simulink model "mySimulationScheme"  (R2021a)
settings: Solver=VariableStepAuto  StartTime=0.0  StopTime=20  RelTol=1e-3
model workspace (MAT data in the model file):
  firstWarning = 1
  originalScenarioChecksum = 'C777D8D004E8227793BA6FB88E4AFE4A'
values from neighbouring files (symbols this model uses):
  A = [0 1 0;0 0 1;0 0 (-1/tau)]    [main.m]
  C = [0 1 0]    [main.m]
  h = 1    [main.m]
  lambda = 50    [main.m]
  Ts = 0.1    [main.m]
undefined symbols (not defined in the file or in its folder): driving, matlabshared
libraries: drivingscenarioandsensors x4, pid_lib x2
(part 1 of 3)
settings Model: EnablePacing=on  PacingRate=0.400000  Creator=nicol  LastModifiedBy=nicol

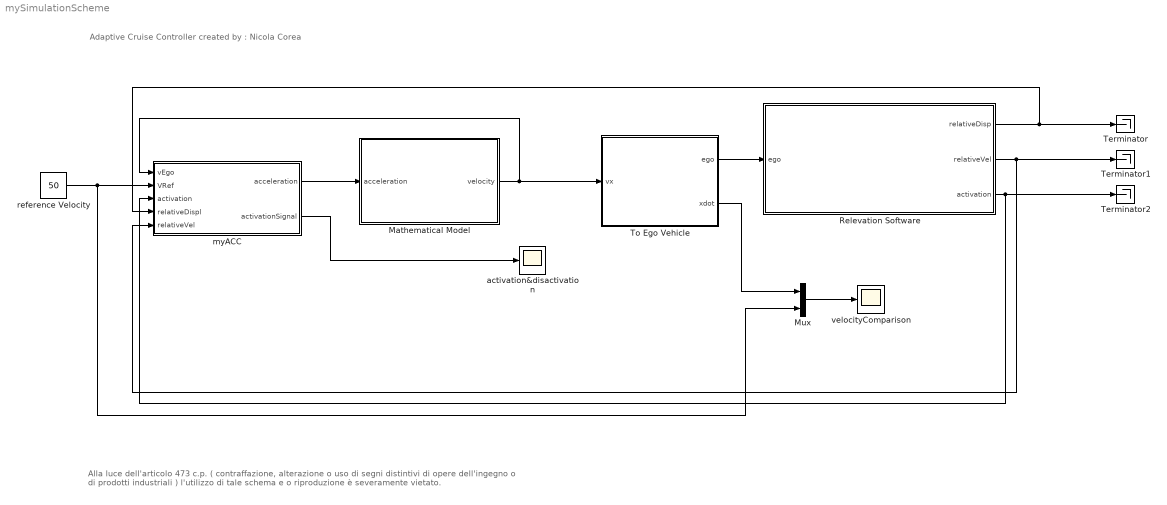
== system mySimulationScheme ==
  note: Alla luce dell'articolo 473 c.p. ( contraffazione, alterazione o uso di segni distintivi di opere dell'ingegno o di prodotti industriali ) l'utilizzo di tale schema e o riproduzione è severamente vietato.
  note: Adaptive Cruise Controller
      | created by : Nicola Corea
  Mathematical Model : Subsystem
  Mux : Mux  Inputs=2
  Relevation Software : Subsystem
  Terminator : Terminator
  Terminator1 : Terminator
  Terminator2 : Terminator
  To Ego Vehicle : Subsystem
  activation&disactivation : Scope
  myACC : Subsystem
  reference Velocity : Constant  Value=50  SampleTime=Ts
  velocityComparison : Scope
  wires:
  Relevation Software/1(relativeDisp) -> myACC/4(relativeDispl), Terminator/1
  Relevation Software/2(relativeVel) -> myACC/5(relativeVel), Terminator1/1
  myACC/1(acceleration) -> Mathematical Model/1(acceleration)
  reference Velocity/1 -> myACC/2(VRef), Mux/2
  Mathematical Model/1(velocity) -> myACC/1(vEgo), To Ego Vehicle/1(vx)
  To Ego Vehicle/1(ego) -> Relevation Software/1(ego)
  To Ego Vehicle/2(xdot) -> Mux/1
  Mux/1 -> velocityComparison/1
  Relevation Software/3(activation) -> myACC/3(activation), Terminator2/1
  myACC/2(activationSignal) -> activation&disactivation/1

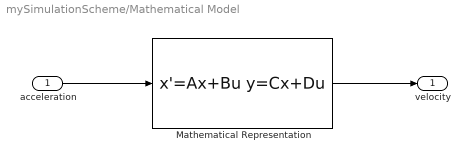
== system mySimulationScheme/Mathematical Model ==
  acceleration : Inport
  Mathematical Representation : StateSpace  A=A  B=B'  C=[0 1 0]  D=0  InitialCondition=0
  velocity : Outport
  wires:
  acceleration/1 -> Mathematical Representation/1
  Mathematical Representation/1 -> velocity/1

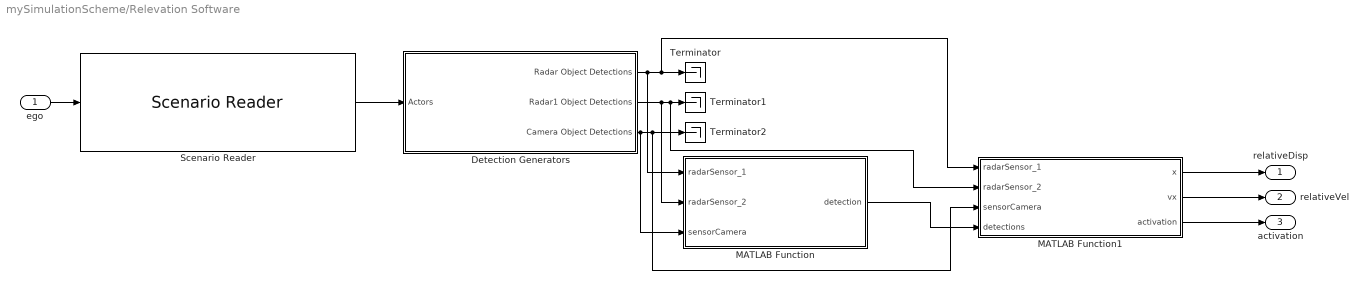
== system mySimulationScheme/Relevation Software ==
  ego : Inport
  Detection Generators : Subsystem
  MATLAB Function : MATLAB Function  TreatAsAtomicUnit=on
  MATLAB Function1 : MATLAB Function  TreatAsAtomicUnit=on
  Scenario Reader : drivingscenarioandsensors/Scenario Reader  ScenarioSource=From file  ScenarioFileName=C:\Users\nicol\Desktop\AdaptiveCruiseControl\myDrivingScenario.mat  ScenarioVariableName=scenario  OutputCoordinateSystem=Vehicle coordinates  EgoVehicleSource=Input port  EgoVehicleActorID=1  OrientVehiclesOnRoad=on  OutputEgoVehiclePose=off  SampleTime=0.1  LaneBoundaryOutput=None  LaneBoundaryDistance=0:0.5:9.5  LaneBoundaryLocation=Center of lane markings  BusNameSource=Auto  BusName=BusActors  BusNumActorsSource=Scenario  BusNumActors=100  BusName2Source=Auto  BusName2=BusLaneBoundaries  BusNumLaneBoundariesSource=Scenario  BusNumLaneBoundaries=10  BusName3Source=Auto  BusName3=BusEgoActor  ShowCoordinateLabels=on  SimulateUsing=Interpreted execution
  Terminator : Terminator
  Terminator1 : Terminator
  Terminator2 : Terminator
  relativeDisp : Outport
  relativeVel : Outport  Port=2
  activation : Outport  Port=3
  wires:
  MATLAB Function1/1(x) -> relativeDisp/1
  Scenario Reader/1 -> Detection Generators/1(Actors)
  MATLAB Function/1(detection) -> MATLAB Function1/4(detections)
  MATLAB Function1/2(vx) -> relativeVel/1
  Detection Generators/1(Radar Object Detections) -> MATLAB Function/1(radarSensor_1), MATLAB Function1/1(radarSensor_1), Terminator/1
  Detection Generators/2(Radar1 Object Detections) -> MATLAB Function/2(radarSensor_2), MATLAB Function1/2(radarSensor_2), Terminator1/1
  Detection Generators/3(Camera Object Detections) -> MATLAB Function/3(sensorCamera), MATLAB Function1/3(sensorCamera), Terminator2/1
  ego/1 -> Scenario Reader/1
  MATLAB Function1/3(activation) -> activation/1

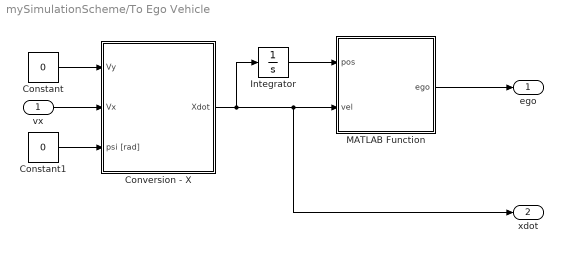
== system mySimulationScheme/To Ego Vehicle ==
  vx : Inport
  Constant : Constant  Value=0
  Constant1 : Constant  Value=0
  Conversion - X : Subsystem
  Integrator : Integrator  InitialCondition=-369.1963
  MATLAB Function : MATLAB Function  TreatAsAtomicUnit=on
  ego : Outport
  xdot : Outport  Port=2
  wires:
  Conversion - X/1(Xdot) -> Integrator/1, xdot/1, MATLAB Function/2(vel)
  Constant/1 -> Conversion - X/1(Vy)
  Constant1/1 -> Conversion - X/3(psi [rad])
  MATLAB Function/1(ego) -> ego/1
  Integrator/1 -> MATLAB Function/1(pos)
  vx/1 -> Conversion - X/2(Vx)

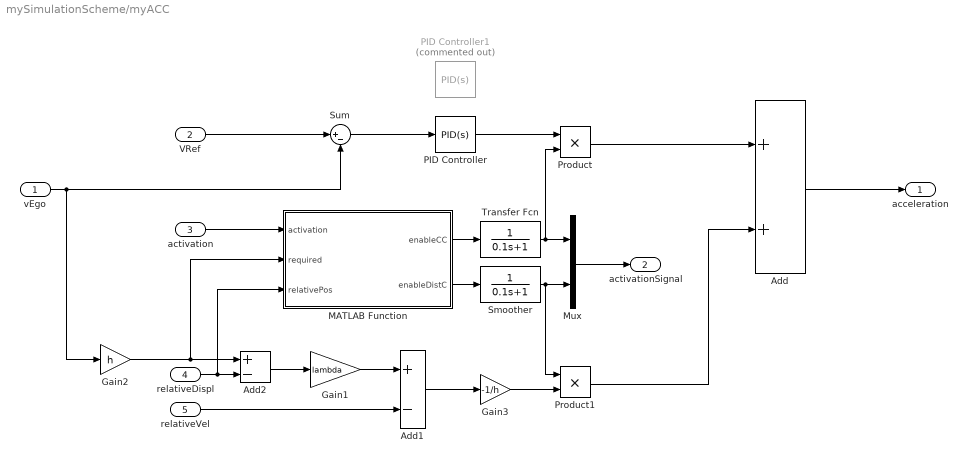
== system mySimulationScheme/myACC ==
  vEgo : Inport
  VRef : Inport  Port=2
  activation : Inport  Port=3
  relativeDispl : Inport  Port=4
  relativeVel : Inport  Port=5
  Add : Sum
  Add1 : Sum  Inputs=+-
  Add2 : Sum  Inputs=+-
  Gain1 : Gain  Gain=lambda
  Gain2 : Gain  Gain=h
  Gain3 : Gain  Gain=-1/h
  MATLAB Function : MATLAB Function  TreatAsAtomicUnit=on
  Mux : Mux  Inputs=2
  PID Controller : pid_lib/PID Controller  Controller=PID  Form=Parallel  TimeDomain=Continuous-time  UseExternalTs=off  SampleTime=-1  IntegratorMethod=Forward Euler  FilterMethod=Forward Euler  ControllerParametersSource=internal  P=4.17595282239104  I=1.94142668336912  D=1.56681262957778  UseFilter=on  N=12.9901005705061  TunerSelectOption=Transfer Function Based (PID Tuner App)  InitialConditionSource=internal  InitialConditionForIntegrator=0  InitialConditionForFilter=0  DifferentiatorICPrevScaledInput=0  ExternalReset=none  TrackingMode=off  Kt=1  LimitOutput=off  SatLimitsSource=internal  UpperSaturationLimit=inf  LowerSaturationLimit=-inf  LinearizeAsGain=on  AntiWindupMode=none  Kb=1  POutMin=[]  POutMax=[]  IOutMin=[]  IOutMax=[]  DOutMin=[]  DOutMax=[]  NOutMin=[]  NOutMax=[]  SumOutMin=[]  SumOutMax=[]  SaturationOutMin=[]  SaturationOutMax=[]  PParamMin=[]  PParamMax=[]  IParamMin=[]  IParamMax=[]  DParamMin=[]  DParamMax=[]  NParamMin=[]  NParamMax=[]  KbParamMin=[]  KbParamMax=[]  KtParamMin=[]  KtParamMax=[]  KbOutMin=[]  KbOutMax=[]  KtOutMin=[]  KtOutMax=[]  IntegratorOutMin=[]  IntegratorOutMax=[]  FilterOutMin=[]  FilterOutMax=[]  SumI1OutMin=[]  SumI1OutMax=[]  SumI2OutMin=[]  SumI2OutMax=[]  SumI3OutMin=[]  SumI3OutMax=[]  SumI4OutMin=[]  SumI4OutMax=[]  SumDOutMin=[]  SumDOutMax=[]  DifferentiatorOutMin=[]  DifferentiatorOutMax=[]  FilterDiffOutCoefMin=[]  FilterDiffOutCoefMax=[]  ReciprocalOutMin=[]  ReciprocalOutMax=[]  SumDenOutMin=[]  SumDenOutMax=[]  SumNumOutMin=[]  SumNumOutMax=[]  DivideOutMin=[]  DivideOutMax=[]  UdiffTsProdOutMin=[]  UdiffTsProdOutMax=[]  NTsProdOutMin=[]  NTsProdOutMax=[]  UintegralTsProdOutMin=[]  UintegralTsProdOutMax=[]  UngainTsProdOutMin=[]  UngainTsProdOutMax=[]  IntegratorContinuousStateAttributes=''  IntegratorStateMustResolveToSignalObject=off  IntegratorRTWStateStorageClass=Auto  FilterContinuousStateAttributes=''  FilterStateMustResolveToSignalObject=off  FilterRTWStateStorageClass=Auto  ParallelPVariant=InternalParameters  IdealPVariant=Disabled  IVariant=InternalParameters  DVariant=InternalParameters  IntegratorVariant=Continuous  SatVariant=Disabled  AWVariant=Passthrough  PCopyVariant=Disabled  TRVariant=Disabled  FdbkBlocksVariant=Forward  IdealPFdbkVariant=Disabled  SatFdbkVariant=Disabled  DerivativeFilterVariant=ContFilter  NVariant=InternalParameters  NCopyVariant=Disabled  FilterICVariant=InternalICsFilter  IntegratorICVariant=InternalICs  ExternalResetVariant=Disabled  TRSumVariant=Passthrough  SumFdbkVariant=Disabled  SumVariant=Sum_PID  TsampFilterVariant=InternalTs  TsampNgainVariant=Passthrough  TsampIntegralVariant=Passthrough  ExternalSaturationOutDataTypeStr=Inherit: Same as second input
  PID Controller1 : pid_lib/PID Controller  Commented=on  Controller=PID  Form=Parallel  TimeDomain=Continuous-time  UseExternalTs=off  SampleTime=-1  IntegratorMethod=Forward Euler  FilterMethod=Forward Euler  ControllerParametersSource=internal  P=49.6181488472629  I=59.2961705052045  D=9.16412581703958  UseFilter=on  N=2136.38029924778  TunerSelectOption=Transfer Function Based (PID Tuner App)  InitialConditionSource=internal  InitialConditionForIntegrator=0  InitialConditionForFilter=0  DifferentiatorICPrevScaledInput=0  ExternalReset=none  TrackingMode=off  Kt=1  LimitOutput=off  SatLimitsSource=internal  UpperSaturationLimit=inf  LowerSaturationLimit=-inf  LinearizeAsGain=on  AntiWindupMode=none  Kb=1  POutMin=[]  POutMax=[]  IOutMin=[]  IOutMax=[]  DOutMin=[]  DOutMax=[]  NOutMin=[]  NOutMax=[]  SumOutMin=[]  SumOutMax=[]  SaturationOutMin=[]  SaturationOutMax=[]  PParamMin=[]  PParamMax=[]  IParamMin=[]  IParamMax=[]  DParamMin=[]  DParamMax=[]  NParamMin=[]  NParamMax=[]  KbParamMin=[]  KbParamMax=[]  KtParamMin=[]  KtParamMax=[]  KbOutMin=[]  KbOutMax=[]  KtOutMin=[]  KtOutMax=[]  IntegratorOutMin=[]  IntegratorOutMax=[]  FilterOutMin=[]  FilterOutMax=[]  SumI1OutMin=[]  SumI1OutMax=[]  SumI2OutMin=[]  SumI2OutMax=[]  SumI3OutMin=[]  SumI3OutMax=[]  SumI4OutMin=[]  SumI4OutMax=[]  SumDOutMin=[]  SumDOutMax=[]  DifferentiatorOutMin=[]  DifferentiatorOutMax=[]  FilterDiffOutCoefMin=[]  FilterDiffOutCoefMax=[]  ReciprocalOutMin=[]  ReciprocalOutMax=[]  SumDenOutMin=[]  SumDenOutMax=[]  SumNumOutMin=[]  SumNumOutMax=[]  DivideOutMin=[]  DivideOutMax=[]  UdiffTsProdOutMin=[]  UdiffTsProdOutMax=[]  NTsProdOutMin=[]  NTsProdOutMax=[]  UintegralTsProdOutMin=[]  UintegralTsProdOutMax=[]  UngainTsProdOutMin=[]  UngainTsProdOutMax=[]  IntegratorContinuousStateAttributes=''  IntegratorStateMustResolveToSignalObject=off  IntegratorRTWStateStorageClass=Auto  FilterContinuousStateAttributes=''  FilterStateMustResolveToSignalObject=off  FilterRTWStateStorageClass=Auto  ParallelPVariant=InternalParameters  IdealPVariant=Disabled  IVariant=InternalParameters  DVariant=InternalParameters  IntegratorVariant=Continuous  SatVariant=Disabled  AWVariant=Passthrough  PCopyVariant=Disabled  TRVariant=Disabled  FdbkBlocksVariant=Forward  IdealPFdbkVariant=Disabled  SatFdbkVariant=Disabled  DerivativeFilterVariant=ContFilter  NVariant=InternalParameters  NCopyVariant=Disabled  FilterICVariant=InternalICsFilter  IntegratorICVariant=InternalICs  ExternalResetVariant=Disabled  TRSumVariant=Passthrough  SumFdbkVariant=Disabled  SumVariant=Sum_PID  TsampFilterVariant=InternalTs  TsampNgainVariant=Passthrough  TsampIntegralVariant=Passthrough  ExternalSaturationOutDataTypeStr=Inherit: Same as second input
  Product : Product
  Product1 : Product
  Smoother : TransferFcn  Denominator=[0.1 1]
  Sum : Sum  Inputs=|+-
  Transfer Fcn : TransferFcn  Denominator=[0.1 1]
  acceleration : Outport
  activationSignal : Outport  Port=2
  wires:
  VRef/1 -> Sum/1
  activation/1 -> MATLAB Function/1(activation)
  Mux/1 -> activationSignal/1
  Product/1 -> Add/1
  Add/1 -> acceleration/1
  Product1/1 -> Add/2
  Transfer Fcn/1 -> Product/2, Mux/1
  MATLAB Function/1(enableCC) -> Transfer Fcn/1
  MATLAB Function/2(enableDistC) -> Smoother/1
  Smoother/1 -> Product1/1, Mux/2
  relativeVel/1 -> Add1/2
  Gain1/1 -> Add1/1
  Add2/1 -> Gain1/1
  relativeDispl/1 -> MATLAB Function/3(relativePos), Add2/2
  vEgo/1 -> Sum/2, Gain2/1
  Gain3/1 -> Product1/2
  Add1/1 -> Gain3/1
  Gain2/1 -> Add2/1, MATLAB Function/2(required)
  PID Controller/1 -> Product/1
  Sum/1 -> PID Controller/1
